simulink model "eml_model_coverage_demo"  (Simulink 6.0)
settings: Solver=ode3  StartTime=0.0  StopTime=1  FixedStep=1  RelTol=1e-3
settings Model: RecordCoverage=on  CovMetricSettings=dcmw  Creator=The MathWorks Inc.  LastModifiedBy=batserve  ExtModeAutoUpdateStatusClock=off  ProdHWDeviceType=Specified
settings DataIOCC: SignalLoggingName=logsOut
settings DebuggingCC: CheckExecutionContextPreStartOutputMsg=on  CheckExecutionContextRuntimeOutputMsg=on  SolverPrmCheckMsg=none
settings HardwareCC: ProdHWDeviceType=Specified

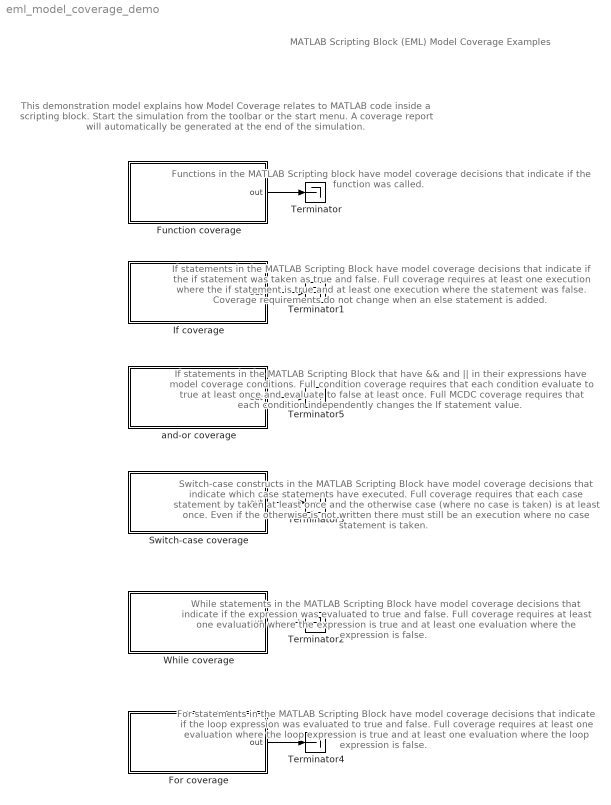
== system eml_model_coverage_demo ==
  note: Functions in the MATLAB Scripting block have model
      | coverage decisions that indicate if the function was called.
  note: MATLAB Scripting Block (EML) Model Coverage Examples
  note: This demonstration model explains how Model Coverage relates
      | to MATLAB code inside a scripting block.
      |
      | Start the simulation from the toolbar or the start menu.  A coverage
      | report will automatically be generated at the end of the simulation.
  note: If statements in the MATLAB Scripting Block have model
      | coverage decisions that indicate if the if statement was taken
      | as true and false.  Full coverage requires at least one
      | execution where the if statement is true and at least one
      | execution where the statement was false.  Coverage
      | requirements do not change when an else statement is added.
  note: Switch-case constructs  in the MATLAB Scripting Block have
      | model coverage decisions that indicate which case statements
      | have executed.  Full coverage requires that each case
      | statement by taken at least once and the otherwise case (where
      | no case is taken) is at least once.  Even if the otherwise
      | is not written there must still be an execution where no case
      | statement is taken.
  note: While statements in the MATLAB Scripting Block have model
      | coverage decisions that indicate if the expression was evaluated
      | to true and false.  Full coverage requires at least one
      | evaluation where the expression is true and at least one
      | evaluation where the expression is false.
  note: For statements in the MATLAB Scripting Block have model
      | coverage decisions that indicate if the loop expression was
      | evaluated to true and false.  Full coverage requires at least one
      | evaluation where the loop expression is true and at least one
      | evaluation where the loop expression is false.
  note: If statements in the MATLAB Scripting Block that have && and ||
      | in their expressions have model coverage conditions.  Full condition
      | coverage requires that each condition evaluate to true at least once
      | and evaluate to false at least once.  Full MCDC coverage requires
      | that each condition independently changes the If statement value.
  For coverage : Stateflow chart  PropExecContextAcrossSSBoundary=on
  Function coverage : Stateflow chart  PropExecContextAcrossSSBoundary=on
  If coverage : Stateflow chart  PropExecContextAcrossSSBoundary=on
  Switch-case coverage : Stateflow chart  PropExecContextAcrossSSBoundary=on
  Terminator{,1..5} (6 alike) : Terminator
  While coverage : Stateflow chart  PropExecContextAcrossSSBoundary=on
  and-or coverage : Stateflow chart  PropExecContextAcrossSSBoundary=on
  wires:
  Function coverage/1(out) -> Terminator/1
  If coverage/1(out) -> Terminator1/1
  While coverage/1(out) -> Terminator2/1
  Switch-case coverage/1(out) -> Terminator3/1
  For coverage/1(out) -> Terminator4/1
  and-or coverage/1(out) -> Terminator5/1

== matlab function If coverage ==
  data: out output double
function out = main
    out = 1;
    out = sub_function(0);
    out = sub_function(1);
    
function out = sub_function(in)
    % An if statement that executes true and false
    if (in==0)
        out = 1;
    else
        out = 2;
    end
    
    % An is statement that is always true
    if (in < 10)
        out = 4;
    end
    
    % An if statement that is always false
    if (in < 0)
        out = 1;
    end

== matlab function Function coverage ==
  data: out output double
function out = main_function
% The main function is called from Simulink
% and is fully covered
    out = 1;
    out = sub_function(2)
    
    
function out = not_called(in)
% This subfunction is not called and is a 
% missing coverage point.
    out = in*2;
    

function out = sub_function(in)
% This subfunction is called from the main
% function and is fully covered
    out = 3*in;

== matlab function While coverage ==
  data: out output double
function out = main
    count = 0;
    out = 1;
    
    % While expression that is always false
    while (count<-1)
        count = count+1;
    end
    
    % While expression that is fully covered
    while (count<5)
        count = count+1;
    end
    
    % While expression that is always true
    while (count < 20)
        count = count+1;
        if (count==10)
            break;
        end
    end
    
    out = count;

== matlab function Switch-case coverage ==
  data: out output double
function out = main
    out = 1;
    out = sub_function(1);
    out = sub_function(2);
    out = sub_function(3);
    
function out = sub_function(in)
    % Fully covered
    switch(in)
    case 1,
        out = 1;
    case 2, 
        out = 2;
    otherwise,
        out = 3;
    end
    
    % Parial coverage (missing "case 4" and implied otherwise)
    switch(in)
    case {1, 2, 3}
        out = 5;
    case 4, 
        out = 6;
    end

== matlab function For coverage ==
  data: out output double
function out = main
    out = 0;
    
    % For expression that is always false
    for idx = 1:out
        out = out+1;
    end
    
    % While expression that is fully covered
    for idx = 1:5
        out = out+1;
    end
    
    % While expression that is always true
    for idx = 1:5
        out = out+1;
        if (idx==3)
            break;
        end
    end

== matlab function and-or coverage ==
  data: out output double
function out = main
    out = 1;
    out = sub_function(0,0);
    out = sub_function(1,0);
    out = sub_function(1,1);
    
function out = sub_function(a,b)
    % Full coverage
    if (a && b)
        out = 1;
    end
    
    % Partial coverage  (1==1 is always True)
    if ( (1==1) && b)
        out = 2;
    end
    
    % Partial coverage (a==b is not True or False)
    if ( a || (~b) || a==b)
        out = 3;
    end
